simulink model "ctrl_sixaxis2force"  (R2015a)
settings: Solver=ode3  StartTime=0.0  StopTime=inf  FixedStep=0.01  RelTol=1e-3
values from neighbouring files (symbols this model uses):
  Max_thrust = 0.12    [initfile.m]
  thrust_to_pwm_coeff = coeffvalues(ForceToPWM)    [initfile.m]
libraries: simulink x3
(part 2 of 2)

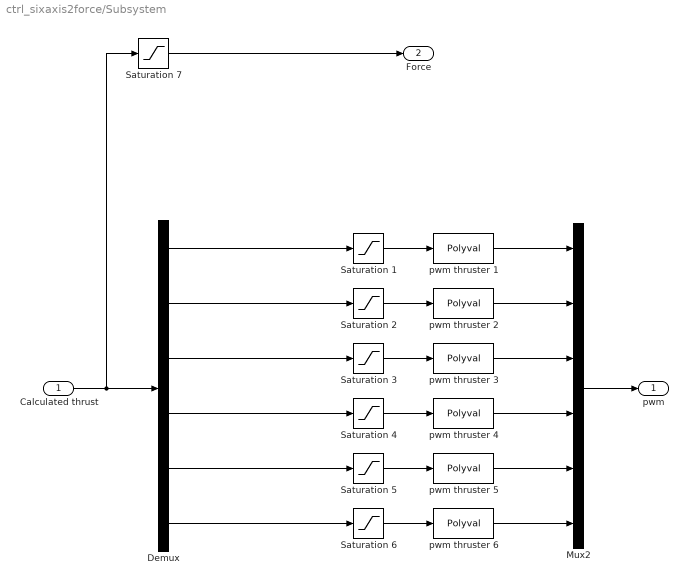
== system ctrl_sixaxis2force/Subsystem ==
  Calculated thrust : Inport
  Demux : Demux  Outputs=6
  Mux2 : Mux  Inputs=6
  Saturation {1..7} (7 alike) : Saturate  UpperLimit=Max_thrust  LowerLimit=-Max_thrust
  pwm thruster {1..6} (6 alike) : Polyval  Coefs=thrust_to_pwm_coeff
  pwm : Outport
  Force : Outport  Port=2
  wires:
  Demux/1 -> Saturation 1/1
  Demux/2 -> Saturation 2/1
  Demux/3 -> Saturation 3/1
  Demux/4 -> Saturation 4/1
  Demux/5 -> Saturation 5/1
  Demux/6 -> Saturation 6/1
  Saturation 1/1 -> pwm thruster 1/1
  Saturation 6/1 -> pwm thruster 6/1
  Saturation 5/1 -> pwm thruster 5/1
  Saturation 4/1 -> pwm thruster 4/1
  Saturation 3/1 -> pwm thruster 3/1
  Saturation 2/1 -> pwm thruster 2/1
  Calculated thrust/1 -> Saturation 7/1, Demux/1
  Mux2/1 -> pwm/1
  pwm thruster 1/1 -> Mux2/1
  pwm thruster 6/1 -> Mux2/6
  pwm thruster 5/1 -> Mux2/5
  pwm thruster 4/1 -> Mux2/4
  pwm thruster 3/1 -> Mux2/3
  pwm thruster 2/1 -> Mux2/2
  Saturation 7/1 -> Force/1

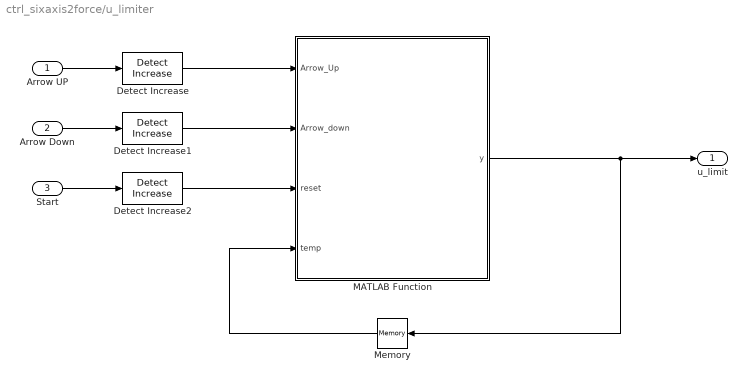
== system ctrl_sixaxis2force/u_limiter ==
  Arrow UP : Inport
  Arrow Down : Inport  Port=2
  Start : Inport  Port=3
  Detect Increase : simulink/Logic and Bit Operations/Detect Increase  vinit=0.0  InputProcessing=Inherited  OutDataTypeStr=boolean
  Detect Increase1 : simulink/Logic and Bit Operations/Detect Increase  vinit=0.0  InputProcessing=Inherited  OutDataTypeStr=boolean
  Detect Increase2 : simulink/Logic and Bit Operations/Detect Increase  vinit=0.0  InputProcessing=Inherited  OutDataTypeStr=boolean
  MATLAB Function : MATLAB Function  TreatAsAtomicUnit=on
  Memory : Memory
  u_limit : Outport
  wires:
  Arrow UP/1 -> Detect Increase/1
  Arrow Down/1 -> Detect Increase1/1
  Memory/1 -> MATLAB Function/4(temp)
  Detect Increase/1 -> MATLAB Function/1(Arrow_Up)
  Detect Increase1/1 -> MATLAB Function/2(Arrow_down)
  Start/1 -> Detect Increase2/1
  Detect Increase2/1 -> MATLAB Function/3(reset)
  MATLAB Function/1(y) -> u_limit/1, Memory/1

== matlab function ctrl_sixaxis2force/Thrust allocation ==
  data: X input; Y input; u_out output; N input; alpha input; body_rel input; alpha_out output; basin_rel input; user_rel input; psi input; user_psi input
function [u_out,alpha_out]= fcn(X,Y,N,alpha,body_rel,basin_rel,user_rel,psi,user_psi)

J = [cos(psi) -sin(psi) 0
     sin(psi) cos(psi)  0
     0        0         1];
 
J_user = [cos(user_psi) -sin(user_psi) 0
     sin(user_psi) cos(user_psi)  0
     0        0         1];

if basin_rel ~= 0
    tc = J*[X,Y,N]';
elseif user_rel ~= 0
    tc = J_user*[X,Y,N]';
elseif body_rel ~= 0
     tc = [X,Y,N]';
else
    tc = [X,Y,N]';
end



Thruster.T1 = [ 96.1/90  0         ];    %[m,m]
Thruster.T2 = [ 89.2/90  9.9/90    ];    %[m,m]
Thruster.T3 = [ 89.2/90 -9.9/90    ];    %[m,m]
Thruster.T4 = [-104.8/90 0         ];    %[m,m] 
Thruster.T5 = [-89.2/90 -14.9/90   ];    %[m,m]
Thruster.T6 = [-89.2/90  14.9/90   ];    %[m,m]
ThrusterPosX = [Thruster.T1(1) Thruster.T2(1) Thruster.T3(1) Thruster.T4(1) Thruster.T5(1) Thruster.T6(1)];%[x(1),x(2),x(3),x(4),x(5),x(6)]';
ThrusterPosY = [Thruster.T1(2) Thruster.T2(2) Thruster.T3(2) Thruster.T4(2) Thruster.T5(2) Thruster.T6(2)];%[x(7),x(8),x(9),x(10),x(11),x(12)]';


n_t = length(ThrusterPosX);

T_surge = zeros(n_t,1); % Shells for faster computing
T_sway = zeros(n_t,1);  % Shells for faster computing
T_yaw = zeros(n_t,1);   % Shells for faster computing

for i = 1:1:n_t
  T_surge(i) = cos(alpha(i));     %Thrust in x-direction for cartesian
  T_sway(i) = sin(alpha(i));      %Thrust in y-direction for cartesian
  T_yaw(i) = (sin(alpha(i))*ThrusterPosX(i) - cos(alpha(i))*ThrusterPosY(i));
end

B = [T_surge,T_sway,T_yaw]';

[U_singular,S_singular,V_singular] = svd(B,'econ');


S_singular_cross = 1./S_singular;
S_singular_cross(~isfinite(S_singular_cross))=0;
 if (S_singular_cross(3,3)>2*S_singular_cross(2,2)) 
     S_singular_cross(3,3)=0;
 end
 
T_optimized = V_singular*S_singular_cross*U_singular';
T_d = T_optimized*tc; 


Te = [1 0 1 0 1 0 1 0 1 0 1 0;
      0 1 0 1 0 1 0 1 0 1 0 1;
      ThrusterPosY(1) ThrusterPosX(1) ThrusterPosY(2) ThrusterPosX(2) ThrusterPosY(3) ThrusterPosX(3) ...
      ThrusterPosY(4) ThrusterPosX(4) ThrusterPosY(5) ThrusterPosX(5) ThrusterPosY(6) ThrusterPosX(6)];
[U_ang,S_ang,V_ang] = svd(Te,'econ');
S_ang = 1./S_ang;
S_ang(~isfinite(S_ang))=0;
 if (S_ang(3,3)>2*S_ang(2,2)) 
     S_ang(3,3)=0;
 end
T0 = V_ang*S_ang*U_ang'*tc;
alpha1 = [atan2(T0(2),T0(1)) atan2(T0(4),T0(3)) atan2(T0(6),T0(5)) atan2(T0(8),T0(7)) atan2(T0(10),T0(9)) atan2(T0(12),T0(11))];

% for i=1:1:n_t
%   if alpha1(i) > 180
%       alpha1(i) = alpha1(i) - 360;
%   elseif alpha1(i) < -180
%       alpha1(i) = alpha1(i) + 360;
%   else
%       alpha1(i);
%   end
% end

u_out = T_d;
alpha_out = alpha1';


end

== matlab function ctrl_sixaxis2force/u_limiter/MATLAB Function ==
  data: Arrow_Up input; y output; Arrow_down input; reset input; temp input
function y = fcn(Arrow_Up,Arrow_down,reset,temp)
%#codegen
persistent signal;

signal = temp;

if Arrow_Up ~= 0
    signal = signal + 0.05;
    
    if signal > 1
        signal = 1;
    end
end

if Arrow_down ~= 0
    signal = signal - 0.05;
    
    if signal < -1
        signal = -1;
    end
end
 
if reset ~= 0
    signal = 0;
end



y = signal;
